simulink model "robotarm_A12_breach"  (R2018b)
settings: Solver=FixedStepAuto  StartTime=0.0  StopTime=tspan(end)  RelTol=1e-3  AbsTol=1e-6
undefined symbols (not defined in the file): options
libraries: neural x132, simulink x2
(part 2 of 6)

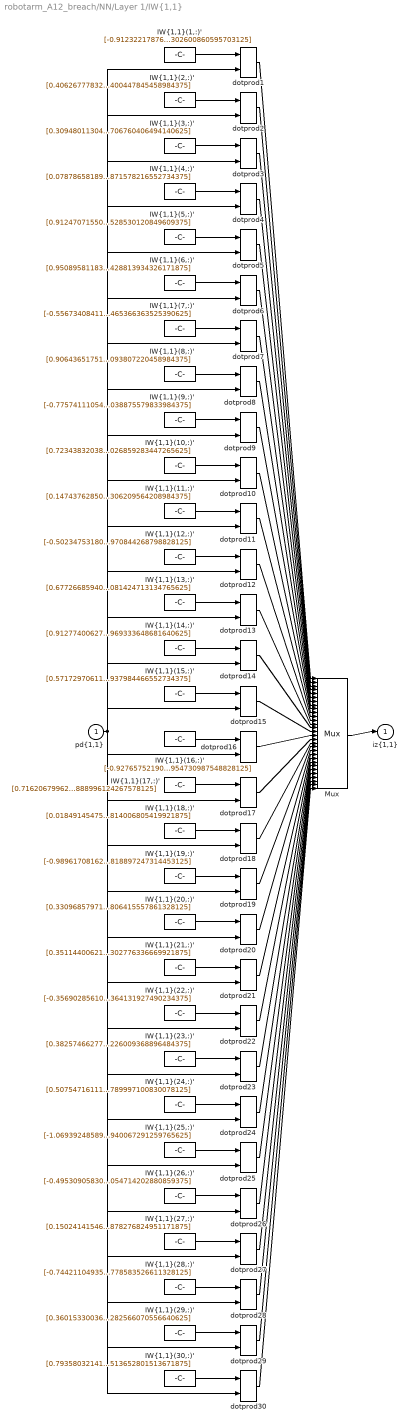
== system robotarm_A12_breach/NN/Layer 1/IW{1,1} ==
  "pd{1,1}" : Inport  PortDimensions=10
      mask Display: e = 0.06;c1 = [120 230 180]/255;c2 = ([120 230 180]+0)/(256+128);c3 = ([120 230 180]+128)/(256+128);patch([0 1 1 0],[0 0 1 1],c1);patch([0 1 1 1-e 1-e 0+e],[0 0 1 1-e 0+e 0+e],c2);patch([0 0 1 1-e 0+e 0+e],[0 1 1 1-e 1-e 0+e],c3);plot([0 1 1 0 0],[0 0 1 1 0]);
  "IW{1,1}(1,:)'" : Constant  Value=[-0.9123221787634481216855419916100800037384033203125;0.34505308101880782789550039524328894913196563720703125;-0.34770242434212217386146903663757257163524627685546875;0.8152839324243055241225874851807020604610443115234375;0.812730198895056599184272272395901381969451904296875;-0.60511073243275836919252697043702937662601470947265625;0.52092599775578296572575709433294832706451416015625;-0.186184222481438232943418142895097844302654266357421875;0.308250067240241787391852312794071622192859649658203125;0.38974914720283149183188697861623950302600860595703125]
      mask Display: e = 0.06;c1 = [120 150 230]/255;c2 = ([120 150 230]+0)/383;c3 = ([120 150 230]+128)/383;patch([0 1 1 0],[0 0 1 1],c1);patch([0 1 1 1-e 1-e 0+e],[0 0 1 1-e 0+e 0+e],c2);patch([0 0 1 1-e 0+e 0+e],[0 1 1 1-e 1-e 0+e],c3);plot([0 1 1 0 0],[0 0 1 1 0]);disp('Weights');
  "IW{1,1}(10,:)'" : Constant  Value=[0.72343832038819499974380278217722661793231964111328125;-0.97016136487421211764825557111180387437343597412109375;0.84434101154705831770996837803977541625499725341796875;-0.55772506778404118410463752297800965607166290283203125;0.47228429165222196584039693334489129483699798583984375;-0.289023516285301707018362549206358380615711212158203125;-0.55341603625618784878525957537931390106678009033203125;-0.3188094529397786924818092302302829921245574951171875;0.254944978839022173833228634975966997444629669189453125;0.42528880133672919416909508072421886026859283447265625]
      mask Display: e = 0.06;c1 = [120 150 230]/255;c2 = ([120 150 230]+0)/383;c3 = ([120 150 230]+128)/383;patch([0 1 1 0],[0 0 1 1],c1);patch([0 1 1 1-e 1-e 0+e],[0 0 1 1-e 0+e 0+e],c2);patch([0 0 1 1-e 0+e 0+e],[0 1 1 1-e 1-e 0+e],c3);plot([0 1 1 0 0],[0 0 1 1 0]);disp('Weights');
  "IW{1,1}(11,:)'" : Constant  Value=[0.1474376285040587541974588248194777406752109527587890625;-0.7769228157862269057432058616541326045989990234375;0.1507471355517946143276475368111277930438518524169921875;0.51492939761651468355552196953794918954372406005859375;-0.69159659449259935914966490599908865988254547119140625;0.7664193792101148261508569703437387943267822265625;-0.86668104946355029039040118732373230159282684326171875;0.366182245298031505686964237611391581594944000244140625;-0.579067202522546065068809184595011174678802490234375;-0.49118402283310957923134765223949216306209564208984375]
      mask Display: e = 0.06;c1 = [120 150 230]/255;c2 = ([120 150 230]+0)/383;c3 = ([120 150 230]+128)/383;patch([0 1 1 0],[0 0 1 1],c1);patch([0 1 1 1-e 1-e 0+e],[0 0 1 1-e 0+e 0+e],c2);patch([0 0 1 1-e 0+e 0+e],[0 1 1 1-e 1-e 0+e],c3);plot([0 1 1 0 0],[0 0 1 1 0]);disp('Weights');
  "IW{1,1}(12,:)'" : Constant  Value=[-0.50234753180376490178105086670257151126861572265625;1.103272598645145041729165313881821930408477783203125;-0.8390687942470582694198810713714919984340667724609375;0.1629024703853648448070856602498679421842098236083984375;-0.031156302752617943963020508135741692967712879180908203125;-0.83268046428062947317272346481331624090671539306640625;0.90892823848490589266901906739803962409496307373046875;-0.1828338801479806596805843810216174460947513580322265625;0.09886895351239644025298503038357011973857879638671875;-0.488358220443266433097306844501872546970844268798828125]
      mask Display: e = 0.06;c1 = [120 150 230]/255;c2 = ([120 150 230]+0)/383;c3 = ([120 150 230]+128)/383;patch([0 1 1 0],[0 0 1 1],c1);patch([0 1 1 1-e 1-e 0+e],[0 0 1 1-e 0+e 0+e],c2);patch([0 0 1 1-e 0+e 0+e],[0 1 1 1-e 1-e 0+e],c3);plot([0 1 1 0 0],[0 0 1 1 0]);disp('Weights');
  "IW{1,1}(13,:)'" : Constant  Value=[0.67726685940645425798578571630059741437435150146484375;-0.84683545365408374738791508207214064896106719970703125;-0.537231642865064973335620379657484591007232666015625;0.037056136714180676339225328774773515760898590087890625;-0.299711915478388990496938504293211735785007476806640625;-0.64977412704210701921425652471953071653842926025390625;0.017207440368440012068429467717578518204391002655029296875;1.0051067512189726382842991370125673711299896240234375;-0.138127211067632871266397387444158084690570831298828125;-0.7750396655798701406325790230766870081424713134765625]
      mask Display: e = 0.06;c1 = [120 150 230]/255;c2 = ([120 150 230]+0)/383;c3 = ([120 150 230]+128)/383;patch([0 1 1 0],[0 0 1 1],c1);patch([0 1 1 1-e 1-e 0+e],[0 0 1 1-e 0+e 0+e],c2);patch([0 0 1 1-e 0+e 0+e],[0 1 1 1-e 1-e 0+e],c3);plot([0 1 1 0 0],[0 0 1 1 0]);disp('Weights');
  "IW{1,1}(14,:)'" : Constant  Value=[0.91277400627938998223243061147513799369335174560546875;-0.232893940901125195974685766486800275743007659912109375;-0.08955948076240143052029196724106441251933574676513671875;0.46842452957560321014085502611123956739902496337890625;-0.1516119293626595199153683779513812623918056488037109375;0.88335999638750439810763737114029936492443084716796875;-0.2407283388399402423996065181199810467660427093505859375;-0.8115003393489403915594948557554744184017181396484375;-0.522724291780654493067004295880906283855438232421875;0.08409965297944511919414622980184503830969333648681640625]
      mask Display: e = 0.06;c1 = [120 150 230]/255;c2 = ([120 150 230]+0)/383;c3 = ([120 150 230]+128)/383;patch([0 1 1 0],[0 0 1 1],c1);patch([0 1 1 1-e 1-e 0+e],[0 0 1 1-e 0+e 0+e],c2);patch([0 0 1 1-e 0+e 0+e],[0 1 1 1-e 1-e 0+e],c3);plot([0 1 1 0 0],[0 0 1 1 0]);disp('Weights');
  "IW{1,1}(15,:)'" : Constant  Value=[0.5717297061163575389031166196218691766262054443359375;-0.917288220020460176584720102255232632160186767578125;0.84265513764526789319830868407734669744968414306640625;-0.93705251740933126480825876569724641740322113037109375;-0.18673810744456142973746182178729213774204254150390625;-0.3789852321320044126196080469526350498199462890625;0.0940124748068315307936160252211266197264194488525390625;0.3594954174353521825224788699415512382984161376953125;-0.63594585456492958019936168057029135525226593017578125;-0.57653312557497338186607294119312427937984466552734375]
      mask Display: e = 0.06;c1 = [120 150 230]/255;c2 = ([120 150 230]+0)/383;c3 = ([120 150 230]+128)/383;patch([0 1 1 0],[0 0 1 1],c1);patch([0 1 1 1-e 1-e 0+e],[0 0 1 1-e 0+e 0+e],c2);patch([0 0 1 1-e 0+e 0+e],[0 1 1 1-e 1-e 0+e],c3);plot([0 1 1 0 0],[0 0 1 1 0]);disp('Weights');
  "IW{1,1}(16,:)'" : Constant  Value=[-0.9276575219077696221603446247172541916370391845703125;-0.8527297494874677141751817543990910053253173828125;0.674357238695943550510492059402167797088623046875;0.7575937746004501871510683486121706664562225341796875;0.44605179816406737014489181092358194291591644287109375;-0.67954350272754660000629201022093184292316436767578125;0.54690913796954154779683676679269410669803619384765625;-0.1749666288236508548958880737700383178889751434326171875;-0.64179505901261768574528332464979030191898345947265625;-0.2185909685816098957378272871210356242954730987548828125]
      mask Display: e = 0.06;c1 = [120 150 230]/255;c2 = ([120 150 230]+0)/383;c3 = ([120 150 230]+128)/383;patch([0 1 1 0],[0 0 1 1],c1);patch([0 1 1 1-e 1-e 0+e],[0 0 1 1-e 0+e 0+e],c2);patch([0 0 1 1-e 0+e 0+e],[0 1 1 1-e 1-e 0+e],c3);plot([0 1 1 0 0],[0 0 1 1 0]);disp('Weights');
  "IW{1,1}(17,:)'" : Constant  Value=[0.7162067996297327709953606245107948780059814453125;0.41942132818541699723624560647294856607913970947265625;-0.79186900108496971473215353398700244724750518798828125;0.735101385621955483173906031879596412181854248046875;-0.72130089412093523204561051898053847253322601318359375;0.70046348646169320772969513200223445892333984375;-0.05417151898146078947693382588113308884203433990478515625;0.09300978554083143279296308492121170274913311004638671875;-0.174357119121888171076051321506383828818798065185546875;-0.86345809789376126719417925414745695888996124267578125]
      mask Display: e = 0.06;c1 = [120 150 230]/255;c2 = ([120 150 230]+0)/383;c3 = ([120 150 230]+128)/383;patch([0 1 1 0],[0 0 1 1],c1);patch([0 1 1 1-e 1-e 0+e],[0 0 1 1-e 0+e 0+e],c2);patch([0 0 1 1-e 0+e 0+e],[0 1 1 1-e 1-e 0+e],c3);plot([0 1 1 0 0],[0 0 1 1 0]);disp('Weights');
  "IW{1,1}(18,:)'" : Constant  Value=[0.0184914547518204262777086199776022112928330898284912109375;0.12280574489549887784445303395841619931161403656005859375;-0.33881203742763077446653596780379302799701690673828125;0.5628854866507106979867103291326202452182769775390625;-1.0511581577404403020636891596950590610504150390625;0.7184653743005282588995896730921231210231781005859375;0.8700974092843221097126615859451703727245330810546875;-0.67805643575585083926426932521280832588672637939453125;-0.0078321107519806233698833608514178195036947727203369140625;0.371484906775879586415811672850395552814006805419921875]
      mask Display: e = 0.06;c1 = [120 150 230]/255;c2 = ([120 150 230]+0)/383;c3 = ([120 150 230]+128)/383;patch([0 1 1 0],[0 0 1 1],c1);patch([0 1 1 1-e 1-e 0+e],[0 0 1 1-e 0+e 0+e],c2);patch([0 0 1 1-e 0+e 0+e],[0 1 1 1-e 1-e 0+e],c3);plot([0 1 1 0 0],[0 0 1 1 0]);disp('Weights');
  "IW{1,1}(19,:)'" : Constant  Value=[-0.98961708162152184353743678002501837909221649169921875;-0.47442181656630488806314360772375948727130889892578125;0.57905987751602328028610600085812620818614959716796875;0.77093936686478292674706835896358825266361236572265625;0.83663846962417476316176134787383489310741424560546875;-1.0137619598726399505750350726884789764881134033203125;0.06545730182129379237654376311184023506939411163330078125;-0.16046184717573785949440434706048108637332916259765625;-0.247131702995537327893771362141706049442291259765625;0.2625615149814866100541621563024818897247314453125]
      mask Display: e = 0.06;c1 = [120 150 230]/255;c2 = ([120 150 230]+0)/383;c3 = ([120 150 230]+128)/383;patch([0 1 1 0],[0 0 1 1],c1);patch([0 1 1 1-e 1-e 0+e],[0 0 1 1-e 0+e 0+e],c2);patch([0 0 1 1-e 0+e 0+e],[0 1 1 1-e 1-e 0+e],c3);plot([0 1 1 0 0],[0 0 1 1 0]);disp('Weights');
  "IW{1,1}(2,:)'" : Constant  Value=[0.40626777832947846835764948991709388792514801025390625;-0.4388444360592729243109033632208593189716339111328125;-0.5377240878110944866108411588356830179691314697265625;-0.637108146502562977531169963185675442218780517578125;0.36525549004092916494101928037707693874835968017578125;-0.60933912729036443511887455315445549786090850830078125;-0.6594475796773988651722220311057753860950469970703125;0.9179232361457156930129031024989672005176544189453125;0.1064490551268389706418560081147006712853908538818359375;-0.60300013933658591636088885934441350400447845458984375]
      mask Display: e = 0.06;c1 = [120 150 230]/255;c2 = ([120 150 230]+0)/383;c3 = ([120 150 230]+128)/383;patch([0 1 1 0],[0 0 1 1],c1);patch([0 1 1 1-e 1-e 0+e],[0 0 1 1-e 0+e 0+e],c2);patch([0 0 1 1-e 0+e 0+e],[0 1 1 1-e 1-e 0+e],c3);plot([0 1 1 0 0],[0 0 1 1 0]);disp('Weights');
  "IW{1,1}(20,:)'" : Constant  Value=[0.330968579712864363617796925609582103788852691650390625;0.6837070431428251549021979371900670230388641357421875;-0.442032416872379319006114428702858276665210723876953125;0.028503968045141707399192654293074156157672405242919921875;0.55511764908762784020979097476811148226261138916015625;-0.53905461219375994108560234963078983128070831298828125;0.88106252350157643338235402552527375519275665283203125;-0.35086862850653688372659644301165826618671417236328125;-0.76683260793421770262767722670105285942554473876953125;-0.64163227196460781431852637979318387806415557861328125]
      mask Display: e = 0.06;c1 = [120 150 230]/255;c2 = ([120 150 230]+0)/383;c3 = ([120 150 230]+128)/383;patch([0 1 1 0],[0 0 1 1],c1);patch([0 1 1 1-e 1-e 0+e],[0 0 1 1-e 0+e 0+e],c2);patch([0 0 1 1-e 0+e 0+e],[0 1 1 1-e 1-e 0+e],c3);plot([0 1 1 0 0],[0 0 1 1 0]);disp('Weights');
  "IW{1,1}(21,:)'" : Constant  Value=[0.351144006212025072688476257098955102264881134033203125;1.0786159452654129342619171438855119049549102783203125;0.72347783244172336747368490250664763152599334716796875;-0.8195873831371314199856215054751373827457427978515625;0.45962340002825763374261214266880415380001068115234375;-0.488261813992200088829775950216571800410747528076171875;0.20425445423965904456764519636635668575763702392578125;-0.1719482276118725894153982380885281600058078765869140625;-0.05798141784361100781186593167149112559854984283447265625;-0.324440372529614773355888246442191302776336669921875]
      mask Display: e = 0.06;c1 = [120 150 230]/255;c2 = ([120 150 230]+0)/383;c3 = ([120 150 230]+128)/383;patch([0 1 1 0],[0 0 1 1],c1);patch([0 1 1 1-e 1-e 0+e],[0 0 1 1-e 0+e 0+e],c2);patch([0 0 1 1-e 0+e 0+e],[0 1 1 1-e 1-e 0+e],c3);plot([0 1 1 0 0],[0 0 1 1 0]);disp('Weights');
  "IW{1,1}(22,:)'" : Constant  Value=[-0.356902856102503107660339765061507932841777801513671875;0.316693863506856965184255159329040907323360443115234375;0.6954494245703444210704446959425695240497589111328125;-0.99427964274322189197619081824086606502532958984375;-0.9794402732072444717204007247346453368663787841796875;0.80403599639925016351327258234960027039051055908203125;0.1406329385698104339486036451489781029522418975830078125;-0.3471812828607008238890330176218412816524505615234375;-0.1537100948899598751307138400079566054046154022216796875;-0.35216615055819155966077005359693430364131927490234375]
      mask Display: e = 0.06;c1 = [120 150 230]/255;c2 = ([120 150 230]+0)/383;c3 = ([120 150 230]+128)/383;patch([0 1 1 0],[0 0 1 1],c1);patch([0 1 1 1-e 1-e 0+e],[0 0 1 1-e 0+e 0+e],c2);patch([0 0 1 1-e 0+e 0+e],[0 1 1 1-e 1-e 0+e],c3);plot([0 1 1 0 0],[0 0 1 1 0]);disp('Weights');
  "IW{1,1}(23,:)'" : Constant  Value=[0.382574662771180296072515147898229770362377166748046875;0.84684434702919630932882455454091541469097137451171875;-0.4386966629716149146389625457231886684894561767578125;-0.9635309885878193814079395451699383556842803955078125;0.27640261224940754214429716739687137305736541748046875;-0.242632556685216493885803856755956076085567474365234375;0.460606365766557501739697499942849390208721160888671875;-0.1594682535722299621117059587049880065023899078369140625;-0.5414567478903611341678470125771127641201019287109375;-0.77980606337009861217524075982510112226009368896484375]
      mask Display: e = 0.06;c1 = [120 150 230]/255;c2 = ([120 150 230]+0)/383;c3 = ([120 150 230]+128)/383;patch([0 1 1 0],[0 0 1 1],c1);patch([0 1 1 1-e 1-e 0+e],[0 0 1 1-e 0+e 0+e],c2);patch([0 0 1 1-e 0+e 0+e],[0 1 1 1-e 1-e 0+e],c3);plot([0 1 1 0 0],[0 0 1 1 0]);disp('Weights');
  "IW{1,1}(24,:)'" : Constant  Value=[0.50754716111374797993249785577063448727130889892578125;0.8334089041544634479663500314927659928798675537109375;-0.2329587095823806297545388588332571089267730712890625;-0.1317275631990683371075334662236855365335941314697265625;0.5060221562888826962733901382307521998882293701171875;0.2067751434713347435945252072997391223907470703125;0.357928903908476259143611741819768212735652923583984375;0.89969115928451603991788942948915064334869384765625;0.5851365243771249335935635826899670064449310302734375;-0.48774768148474401119329968423699028789997100830078125]
      mask Display: e = 0.06;c1 = [120 150 230]/255;c2 = ([120 150 230]+0)/383;c3 = ([120 150 230]+128)/383;patch([0 1 1 0],[0 0 1 1],c1);patch([0 1 1 1-e 1-e 0+e],[0 0 1 1-e 0+e 0+e],c2);patch([0 0 1 1-e 0+e 0+e],[0 1 1 1-e 1-e 0+e],c3);plot([0 1 1 0 0],[0 0 1 1 0]);disp('Weights');
  "IW{1,1}(25,:)'" : Constant  Value=[-1.0693924858933987476206084465957246720790863037109375;0.309190865427156291733723492143326438963413238525390625;0.044860115002628785096927543918354786001145839691162109375;0.9211025006680630955457900199689902365207672119140625;-0.336538787983151455041053168315556831657886505126953125;0.9882203856831213162337235189625062048435211181640625;0.35082830948610099763840253217495046555995941162109375;-0.59001853061985254367272091258200816810131072998046875;-0.27301819039594954485750122330500744283199310302734375;0.10296834613252538181971118547153309918940067291259765625]
      mask Display: e = 0.06;c1 = [120 150 230]/255;c2 = ([120 150 230]+0)/383;c3 = ([120 150 230]+128)/383;patch([0 1 1 0],[0 0 1 1],c1);patch([0 1 1 1-e 1-e 0+e],[0 0 1 1-e 0+e 0+e],c2);patch([0 0 1 1-e 0+e 0+e],[0 1 1 1-e 1-e 0+e],c3);plot([0 1 1 0 0],[0 0 1 1 0]);disp('Weights');
  "IW{1,1}(26,:)'" : Constant  Value=[-0.49530905830905458397950269500142894685268402099609375;0.60143715314780676894912403440685011446475982666015625;0.7338734340457062632623319586855359375476837158203125;-0.61092581403898549297082354314625263214111328125;0.046229710672656264269786419163210666738450527191162109375;-0.63218878527184119153758956599631346762180328369140625;0.82801149438901011645697280982858501374721527099609375;0.543467070792797102285476285032927989959716796875;-0.52772717644786826252101263889926485717296600341796875;0.71693031518041505645300048854551278054714202880859375]
      mask Display: e = 0.06;c1 = [120 150 230]/255;c2 = ([120 150 230]+0)/383;c3 = ([120 150 230]+128)/383;patch([0 1 1 0],[0 0 1 1],c1);patch([0 1 1 1-e 1-e 0+e],[0 0 1 1-e 0+e 0+e],c2);patch([0 0 1 1-e 0+e 0+e],[0 1 1 1-e 1-e 0+e],c3);plot([0 1 1 0 0],[0 0 1 1 0]);disp('Weights');
  "IW{1,1}(27,:)'" : Constant  Value=[0.15024141546899716370688793176668696105480194091796875;0.332395940105069065406695472120190970599651336669921875;-0.84575624494140988485213483727420680224895477294921875;-0.5171856281865865323510433881892822682857513427734375;0.18545836983829910860066547684255056083202362060546875;-0.585103204644562335801083463593386113643646240234375;1.042694219198372795887053143815137445926666259765625;-0.6045617017945608129281254150555469095706939697265625;0.8056948875724605496628782930201850831508636474609375;-0.135567335884474615692596444205264560878276824951171875]
      mask Display: e = 0.06;c1 = [120 150 230]/255;c2 = ([120 150 230]+0)/383;c3 = ([120 150 230]+128)/383;patch([0 1 1 0],[0 0 1 1],c1);patch([0 1 1 1-e 1-e 0+e],[0 0 1 1-e 0+e 0+e],c2);patch([0 0 1 1-e 0+e 0+e],[0 1 1 1-e 1-e 0+e],c3);plot([0 1 1 0 0],[0 0 1 1 0]);disp('Weights');
  "IW{1,1}(28,:)'" : Constant  Value=[-0.74421104935652759859721072643878869712352752685546875;0.8389393286576265484910663872142322361469268798828125;0.8554151355308230453289297656738199293613433837890625;-0.88385262808725284511268682763329707086086273193359375;-0.0754802493071297375681893981891334988176822662353515625;-0.2170881869302884459305147402119473554193973541259765625;-0.07716610542789408000441397916802088730037212371826171875;-0.37622874957520913152819730385090224444866180419921875;-0.0804032721350493029266459643622511066496372222900390625;-0.79469419915195971260146734493901021778583526611328125]
      mask Display: e = 0.06;c1 = [120 150 230]/255;c2 = ([120 150 230]+0)/383;c3 = ([120 150 230]+128)/383;patch([0 1 1 0],[0 0 1 1],c1);patch([0 1 1 1-e 1-e 0+e],[0 0 1 1-e 0+e 0+e],c2);patch([0 0 1 1-e 0+e 0+e],[0 1 1 1-e 1-e 0+e],c3);plot([0 1 1 0 0],[0 0 1 1 0]);disp('Weights');
  "IW{1,1}(29,:)'" : Constant  Value=[0.360153300361462758161223973729647696018218994140625;-0.486055754073548229587942159923841245472431182861328125;0.56845753247753094683503150008618831634521484375;-0.26396991658863011576130475077661685645580291748046875;-0.258208968398081661899112759783747605979442596435546875;-0.7044109842523449405149449376040138304233551025390625;0.2240241320587047224588417293489328585565090179443359375;0.4812551022673605682911102121579460799694061279296875;0.95841705949603295255911916683544404804706573486328125;0.95146335287465577668086780249723233282566070556640625]
      mask Display: e = 0.06;c1 = [120 150 230]/255;c2 = ([120 150 230]+0)/383;c3 = ([120 150 230]+128)/383;patch([0 1 1 0],[0 0 1 1],c1);patch([0 1 1 1-e 1-e 0+e],[0 0 1 1-e 0+e 0+e],c2);patch([0 0 1 1-e 0+e 0+e],[0 1 1 1-e 1-e 0+e],c3);plot([0 1 1 0 0],[0 0 1 1 0]);disp('Weights');
  "IW{1,1}(3,:)'" : Constant  Value=[0.309480113040625115505832809503772296011447906494140625;-0.09919183428964910287373157871115836314857006072998046875;-0.08770973407430039670007460017586709000170230865478515625;0.375423573027454271500147342521813698112964630126953125;-0.8366579862657135269188302117981947958469390869140625;0.759780147842203934516192020964808762073516845703125;0.93942347242478951852007185152615420520305633544921875;-0.495050753676027299743367393602966330945491790771484375;-0.3695518875524523849662728025577962398529052734375;0.75586494997990671951271224315860308706760406494140625]
      mask Display: e = 0.06;c1 = [120 150 230]/255;c2 = ([120 150 230]+0)/383;c3 = ([120 150 230]+128)/383;patch([0 1 1 0],[0 0 1 1],c1);patch([0 1 1 1-e 1-e 0+e],[0 0 1 1-e 0+e 0+e],c2);patch([0 0 1 1-e 0+e 0+e],[0 1 1 1-e 1-e 0+e],c3);plot([0 1 1 0 0],[0 0 1 1 0]);disp('Weights');
  "IW{1,1}(30,:)'" : Constant  Value=[0.7935803214177845621435380962793715298175811767578125;-0.7670489483230820138004446562263183295726776123046875;0.20107215321500870874871225169044919312000274658203125;0.1575830537383592633293716289699659682810306549072265625;-0.69946391073995550780040275640203617513179779052734375;0.12735133891807404182827667682431638240814208984375;-0.10823148190044895589068119079456664621829986572265625;-0.71907657708865091450434192665852606296539306640625;-0.8348790756931594447820543791749514639377593994140625;0.207672402442691861335077874173293821513652801513671875]
      mask Display: e = 0.06;c1 = [120 150 230]/255;c2 = ([120 150 230]+0)/383;c3 = ([120 150 230]+128)/383;patch([0 1 1 0],[0 0 1 1],c1);patch([0 1 1 1-e 1-e 0+e],[0 0 1 1-e 0+e 0+e],c2);patch([0 0 1 1-e 0+e 0+e],[0 1 1 1-e 1-e 0+e],c3);plot([0 1 1 0 0],[0 0 1 1 0]);disp('Weights');
  "IW{1,1}(4,:)'" : Constant  Value=[0.0787865818932858841261435145497671328485012054443359375;0.2101023468095224444596169632859528064727783203125;-0.75002183916029985244477984451805241405963897705078125;0.94576667751902598890723083968623541295528411865234375;-0.6447201953804821972227045989711768925189971923828125;0.38657798541537113923283186522894538938999176025390625;-1.01974497659164686780286501743830740451812744140625;0.760161455931125384921642762492410838603973388671875;0.03132429587165579121244007865243474952876567840576171875;0.339059428884775027057685292675159871578216552734375]
      mask Display: e = 0.06;c1 = [120 150 230]/255;c2 = ([120 150 230]+0)/383;c3 = ([120 150 230]+128)/383;patch([0 1 1 0],[0 0 1 1],c1);patch([0 1 1 1-e 1-e 0+e],[0 0 1 1-e 0+e 0+e],c2);patch([0 0 1 1-e 0+e 0+e],[0 1 1 1-e 1-e 0+e],c3);plot([0 1 1 0 0],[0 0 1 1 0]);disp('Weights');
  "IW{1,1}(5,:)'" : Constant  Value=[0.912470715502206264346796160680241882801055908203125;0.06052545416144512746559058768980321474373340606689453125;0.91822533181494225829055721987970173358917236328125;-0.37304142735173773104406791389919817447662353515625;0.2300422438979922989954474132900941185653209686279296875;-0.348860673310405433600323021892108954489231109619140625;-0.2358519155655350030276196093836915679275989532470703125;-0.445719358726977044060646448997431434690952301025390625;0.84215647381733571563700024853460490703582763671875;-0.3047843207901512752044936860329471528530120849609375]
      mask Display: e = 0.06;c1 = [120 150 230]/255;c2 = ([120 150 230]+0)/383;c3 = ([120 150 230]+128)/383;patch([0 1 1 0],[0 0 1 1],c1);patch([0 1 1 1-e 1-e 0+e],[0 0 1 1-e 0+e 0+e],c2);patch([0 0 1 1-e 0+e 0+e],[0 1 1 1-e 1-e 0+e],c3);plot([0 1 1 0 0],[0 0 1 1 0]);disp('Weights');
  "IW{1,1}(6,:)'" : Constant  Value=[0.950895811834726600864087231457233428955078125;-0.25173201043532078546860475398716516792774200439453125;0.358504972604424543280998705085949040949344635009765625;-0.53012079456372307451061942629166878759860992431640625;-0.290305739557548403428910432921838946640491485595703125;0.86599502732583089059659187114448286592960357666015625;-0.164957864157337652510904035807470791041851043701171875;0.60844500488736696919289670404396019876003265380859375;-0.66036216299820449382451670317095704376697540283203125;0.75806252597195011855291113533894531428813934326171875]
      mask Display: e = 0.06;c1 = [120 150 230]/255;c2 = ([120 150 230]+0)/383;c3 = ([120 150 230]+128)/383;patch([0 1 1 0],[0 0 1 1],c1);patch([0 1 1 1-e 1-e 0+e],[0 0 1 1-e 0+e 0+e],c2);patch([0 0 1 1-e 0+e 0+e],[0 1 1 1-e 1-e 0+e],c3);plot([0 1 1 0 0],[0 0 1 1 0]);disp('Weights');
  "IW{1,1}(7,:)'" : Constant  Value=[-0.55673408411787550509330912973382510244846343994140625;-0.76725817052760447722903336398303508758544921875;-0.2332800862419021903360061287457938306033611297607421875;0.340215575082592369682288335752673447132110595703125;-1.056933352435454498419176161405630409717559814453125;0.336009940701773868187984817268443293869495391845703125;0.99009452197866931744130170045536942780017852783203125;-0.1568706652775886112305414599177311174571514129638671875;-0.002028040969732173952333464939101759227924048900604248046875;0.1041510266466333656243392624674015678465366363525390625]
      mask Display: e = 0.06;c1 = [120 150 230]/255;c2 = ([120 150 230]+0)/383;c3 = ([120 150 230]+128)/383;patch([0 1 1 0],[0 0 1 1],c1);patch([0 1 1 1-e 1-e 0+e],[0 0 1 1-e 0+e 0+e],c2);patch([0 0 1 1-e 0+e 0+e],[0 1 1 1-e 1-e 0+e],c3);plot([0 1 1 0 0],[0 0 1 1 0]);disp('Weights');
  "IW{1,1}(8,:)'" : Constant  Value=[0.9064365175126010143458188395015895366668701171875;-0.435469426069328646722311759731383062899112701416015625;-0.4197081705497602843735194255714304745197296142578125;-0.26196364044401942994255705343675799667835235595703125;-0.96163758896771833750705127386027015745639801025390625;0.1874988806951601028050191644069855101406574249267578125;0.76285817558765411927623745214077644050121307373046875;0.314771325320255701551985794139909557998180389404296875;0.74717657010645288639949512798921205103397369384765625;-0.20891309565003179926634402363561093807220458984375]
      mask Display: e = 0.06;c1 = [120 150 230]/255;c2 = ([120 150 230]+0)/383;c3 = ([120 150 230]+128)/383;patch([0 1 1 0],[0 0 1 1],c1);patch([0 1 1 1-e 1-e 0+e],[0 0 1 1-e 0+e 0+e],c2);patch([0 0 1 1-e 0+e 0+e],[0 1 1 1-e 1-e 0+e],c3);plot([0 1 1 0 0],[0 0 1 1 0]);disp('Weights');
  "IW{1,1}(9,:)'" : Constant  Value=[-0.775741110544188483544303380767814815044403076171875;-0.2739259816727095397936864173971116542816162109375;0.037519492314415751887946015585839631967246532440185546875;0.9639979993417477910355728454305790364742279052734375;-0.10210000679444776461313182380763464607298374176025390625;0.209363900906797406609172185198985971510410308837890625;0.322054355184262786071514028662932105362415313720703125;-0.66755083054416941568121046657324768602848052978515625;-0.694750263960344227598397992551326751708984375;0.9279735465101823788103274637251161038875579833984375]
      mask Display: e = 0.06;c1 = [120 150 230]/255;c2 = ([120 150 230]+0)/383;c3 = ([120 150 230]+128)/383;patch([0 1 1 0],[0 0 1 1],c1);patch([0 1 1 1-e 1-e 0+e],[0 0 1 1-e 0+e 0+e],c2);patch([0 0 1 1-e 0+e 0+e],[0 1 1 1-e 1-e 0+e],c3);plot([0 1 1 0 0],[0 0 1 1 0]);disp('Weights');
  Mux : Mux  Inputs=30
      mask Display: e = 0.06;c1 = [120 150 230]/255;c2 = ([120 150 230]+0)/383;c3 = ([120 150 230]+128)/383;patch([0 1 1 0],[0 0 1 1],c1);patch([0 1 1 1-e 1-e 0+e],[0 0 1 1-e 0+e 0+e],c2);patch([0 0 1 1-e 0+e 0+e],[0 1 1 1-e 1-e 0+e],c3);plot([0 1 1 0 0],[0 0 1 1 0]);disp('Mux');
  dotprod{1..30} (30 alike) : neural/Weight Functions/dotprod
  "iz{1,1}" : Outport
      mask Display: e = 0.06;c1 = [120 230 180]/255;c2 = ([120 230 180]+0)/(256+128);c3 = ([120 230 180]+128)/(256+128);patch([0 1 1 0],[0 0 1 1],c1);patch([0 1 1 1-e 1-e 0+e],[0 0 1 1-e 0+e 0+e],c2);patch([0 0 1 1-e 0+e 0+e],[0 1 1 1-e 1-e 0+e],c3);plot([0 1 1 0 0],[0 0 1 1 0]);
  wires:
  "IW{1,1}(1,:)'"/1 -> dotprod1/1
  "pd{1,1}"/1 -> dotprod1/2, dotprod2/2, dotprod3/2, dotprod4/2, dotprod5/2, dotprod6/2, dotprod7/2, dotprod8/2, dotprod9/2, dotprod10/2, dotprod11/2, dotprod12/2, dotprod13/2, dotprod14/2, dotprod15/2, dotprod16/2, dotprod17/2, dotprod18/2, dotprod19/2, dotprod20/2, dotprod21/2, dotprod22/2, dotprod23/2, dotprod24/2, dotprod25/2, dotprod26/2, dotprod27/2, dotprod28/2, dotprod29/2, dotprod30/2
  dotprod1/1 -> Mux/1
  "IW{1,1}(2,:)'"/1 -> dotprod2/1
  dotprod2/1 -> Mux/2
  "IW{1,1}(3,:)'"/1 -> dotprod3/1
  dotprod3/1 -> Mux/3
  "IW{1,1}(4,:)'"/1 -> dotprod4/1
  dotprod4/1 -> Mux/4
  "IW{1,1}(5,:)'"/1 -> dotprod5/1
  dotprod5/1 -> Mux/5
  "IW{1,1}(6,:)'"/1 -> dotprod6/1
  dotprod6/1 -> Mux/6
  "IW{1,1}(7,:)'"/1 -> dotprod7/1
  dotprod7/1 -> Mux/7
  "IW{1,1}(8,:)'"/1 -> dotprod8/1
  dotprod8/1 -> Mux/8
  "IW{1,1}(9,:)'"/1 -> dotprod9/1
  dotprod9/1 -> Mux/9
  "IW{1,1}(10,:)'"/1 -> dotprod10/1
  dotprod10/1 -> Mux/10
  "IW{1,1}(11,:)'"/1 -> dotprod11/1
  dotprod11/1 -> Mux/11
  "IW{1,1}(12,:)'"/1 -> dotprod12/1
  dotprod12/1 -> Mux/12
  "IW{1,1}(13,:)'"/1 -> dotprod13/1
  dotprod13/1 -> Mux/13
  "IW{1,1}(14,:)'"/1 -> dotprod14/1
  dotprod14/1 -> Mux/14
  "IW{1,1}(15,:)'"/1 -> dotprod15/1
  dotprod15/1 -> Mux/15
  "IW{1,1}(16,:)'"/1 -> dotprod16/1
  dotprod16/1 -> Mux/16
  "IW{1,1}(17,:)'"/1 -> dotprod17/1
  dotprod17/1 -> Mux/17
  "IW{1,1}(18,:)'"/1 -> dotprod18/1
  dotprod18/1 -> Mux/18
  "IW{1,1}(19,:)'"/1 -> dotprod19/1
  dotprod19/1 -> Mux/19
  "IW{1,1}(20,:)'"/1 -> dotprod20/1
  dotprod20/1 -> Mux/20
  "IW{1,1}(21,:)'"/1 -> dotprod21/1
  dotprod21/1 -> Mux/21
  "IW{1,1}(22,:)'"/1 -> dotprod22/1
  dotprod22/1 -> Mux/22
  "IW{1,1}(23,:)'"/1 -> dotprod23/1
  dotprod23/1 -> Mux/23
  "IW{1,1}(24,:)'"/1 -> dotprod24/1
  dotprod24/1 -> Mux/24
  "IW{1,1}(25,:)'"/1 -> dotprod25/1
  dotprod25/1 -> Mux/25
  "IW{1,1}(26,:)'"/1 -> dotprod26/1
  dotprod26/1 -> Mux/26
  "IW{1,1}(27,:)'"/1 -> dotprod27/1
  dotprod27/1 -> Mux/27
  "IW{1,1}(28,:)'"/1 -> dotprod28/1
  dotprod28/1 -> Mux/28
  "IW{1,1}(29,:)'"/1 -> dotprod29/1
  dotprod29/1 -> Mux/29
  "IW{1,1}(30,:)'"/1 -> dotprod30/1
  dotprod30/1 -> Mux/30
  Mux/1 -> "iz{1,1}"/1

== system robotarm_A12_breach/NN/Layer 2/Delays 1 ==
  "p{2}" : Inport  PortDimensions=30
      mask Display: e = 0.06;c1 = [120 230 180]/255;c2 = ([120 230 180]+0)/(256+128);c3 = ([120 230 180]+128)/(256+128);patch([0 1 1 0],[0 0 1 1],c1);patch([0 1 1 1-e 1-e 0+e],[0 0 1 1-e 0+e 0+e],c2);patch([0 0 1 1-e 0+e 0+e],[0 1 1 1-e 1-e 0+e],c3);plot([0 1 1 0 0],[0 0 1 1 0]);
  mux : Mux  Inputs=1
      mask Display: e = 0.06;c1 = [120 150 230]/255;c2 = ([120 150 230]+0)/383;c3 = ([120 150 230]+128)/383;patch([0 1 1 0],[0 0 1 1],c1);patch([0 1 1 1-e 1-e 0+e],[0 0 1 1-e 0+e 0+e],c2);patch([0 0 1 1-e 0+e 0+e],[0 1 1 1-e 1-e 0+e],c3);plot([0 1 1 0 0],[0 0 1 1 0]);disp('Mux')
  "pd{2,1}" : Outport
      mask Display: e = 0.06;c1 = [120 230 180]/255;c2 = ([120 230 180]+0)/(256+128);c3 = ([120 230 180]+128)/(256+128);patch([0 1 1 0],[0 0 1 1],c1);patch([0 1 1 1-e 1-e 0+e],[0 0 1 1-e 0+e 0+e],c2);patch([0 0 1 1-e 0+e 0+e],[0 1 1 1-e 1-e 0+e],c3);plot([0 1 1 0 0],[0 0 1 1 0]);
  wires:
  "p{2}"/1 -> mux/1
  mux/1 -> "pd{2,1}"/1
